simulink model "eVTOL_3DVisuals"  (R2024a)
settings: Solver=VariableStepAuto  StartTime=0.0  StopTime=inf  RelTol=1e-3
libraries: etargetslib x3, slrealtimeiplib x3, sim3dlib x1, uavsim3dlib x1, uavutilslib x1
settings Model: DataDictionary=VTOLDynamicsData.sldd  Creator=jatin.anand  LastModifiedBy=jatin.anand

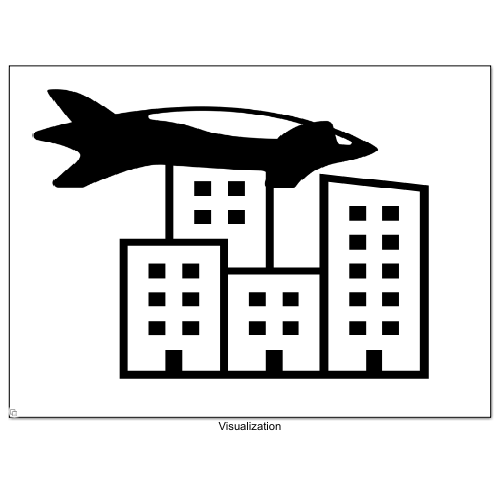
[thumbnail: Simulink's stored preview of the top-level diagram]
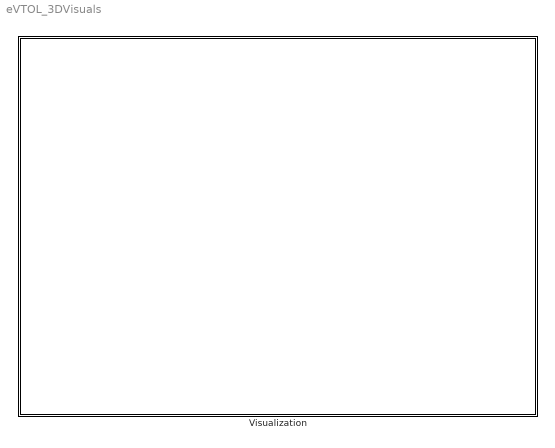
== system eVTOL_3DVisuals ==
  Visualization : Subsystem  Variant=on  VariantControl=Visualization
      mask Display: image('3DVisualization.png');

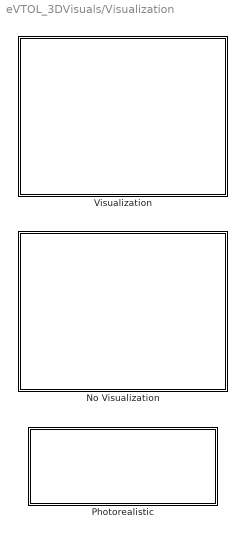
== system eVTOL_3DVisuals/Visualization ==
  No Visualization : Subsystem  VariantControl=Visualization==0
  Photorealistic : Subsystem  VariantControl=Visualization==2
  Visualization : Subsystem  VariantControl=Visualization==1

== system eVTOL_3DVisuals/Visualization/No Visualization ==

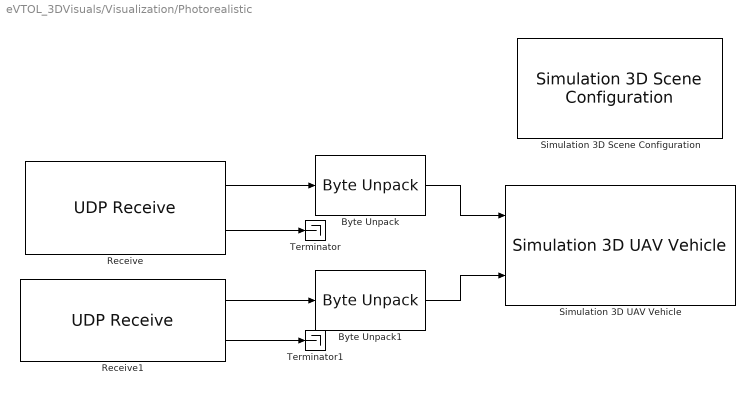
== system eVTOL_3DVisuals/Visualization/Photorealistic ==
  Byte Unpack : etargetslib/Byte Unpack  dimensions={[3]}  datatypes={'double'}  byteAlign=1
      settings: LibrarySourceBlock=embeddedtargetslib/Host Communication/Byte Unpack
  Byte Unpack1 : etargetslib/Byte Unpack  dimensions={[3]}  datatypes={'double'}  byteAlign=1
      settings: LibrarySourceBlock=embeddedtargetslib/Host Communication/Byte Unpack
  Receive : slrealtimeiplib/UDP Receive  useHostTargetConn=on  ipAddress=target_ip  localPort=25002  rcvWidth=24  rcvFmAny=on  fmAddress=host_ip  sampleTime=-1  enableMessage=off  maxPackets=1
  Receive1 : slrealtimeiplib/UDP Receive  useHostTargetConn=on  ipAddress=target_ip  localPort=25003  rcvWidth=24  rcvFmAny=on  fmAddress=host_ip  sampleTime=-1  enableMessage=off  maxPackets=1
  Simulation 3D Scene Configuration : sim3dlib/Simulation 3D Scene Configuration  Priority=0  ProjectFormat=Unreal Editor  SceneDesc=US city block  ProjectName=I:\29\vdubey.MergedFixedWingReview\matlab\toolbox\shared\sim3d_projects\automotive_project_windows\UE\WindowsNoEditor\VehicleSimulation.exe  ScenePath=/Game/Maps/USCityBlock  UEProjPath=C:\project\AutoVrtlEnv\AutoVrtlEnv.uproject  EnableOpenDRIVE=off  vehTagList={'Scene Origin'}  vehTag=Scene Origin  FreeCameraInitialTranslation=[0, 0, 0]  FreeCameraDefaultInitialTranslation=[-6, 0, 2]  FreeCameraInitialRotation=[0, 0, 0]  FreeCameraDefaultInitialRotation=[0, -15, 0]  OpVisEn=off  Ts=1/10  EnableWindow=on  EnableRemoteAccess=off  EnableWeather=off  SunAzimuth=90  SunAltitude=40.0  EnableGeospatialSun=off  Latitude=0  Longitude=0  Date=2023-01-01  Time=10:30:00  GeoTimeZone=-5.0  SunDaylightSaving=off  wind=1  clouds=10  EnableVolumetricClouds=off  CloudCoverage=0  CloudAltitude=6  fog=0  rain=0  RaindropsEffect=off  SnowDensity=0  EnableGeospatial=off  UseTrueOrigin=off  OriginHeight=200  OriginLatitude=40.744652  OriginLongitude=-73.988864  MapStyle=Aerial  AdditionalAssetIDs=[]  UseAdvancedSunSky=off  SolarTime=11  TimeZone=-5  Day=21  Month=9  Year=2022  UseDaylightSavingTime=on  DSTStartDay=10  DSTStartMonth=3  DSTEndDay=3  DSTEndMonth=11  DSTSwitchHour=2  sensorTag=MainCamera1  sensorId=1  sensorName=MainCamera1  mountLoc=Origin  offsetFlag=off  tmountOffset=[0, 0, 0]  rmountOffset=[0, 0, 0]  HorizontalResolution=1280  VerticalResolution=720  HorizontalFOV=60  mountPoint=[0 0 0]  mountOrientation=[0 0 0]  aMode=4  ID=1  GeoTrigger=Inactive
      link override Simulation 3D Engine: SceneDesc=US city block
      settings: LibrarySourceBlock=uavsim3dlib/Simulation 3D Scene Configuration
  Simulation 3D UAV Vehicle : uavsim3dlib/Simulation 3D UAV Vehicle  Priority=-1  Mesh=Custom  MeshPath=SkeletalMesh'/Game/Maps/VTOLDEMO/VTOLAsset.VTOLAsset'  Color=Black  ActorName=SimulinkVehicle1  UseGlobalFrame=off  InitialTranslation=[0 0 0]  InitialRotation=[0 0 0]  InitialTranslationGlobal=[0 0 0]  InitialGeoOrigin=[0 0 0]  InitialRotationGlobal=[0 0 0]  SampleTime=0.1  ActorType=SimulinkVehicle  ID=1  aMode=4  ActorTag=SimulinkVehicle1
  Terminator : Terminator
  Terminator1 : Terminator
  wires:
  Receive1/1 -> Byte Unpack1/1
  Receive/1 -> Byte Unpack/1
  Receive/2 -> Terminator/1
  Receive1/2 -> Terminator1/1
  Byte Unpack/1 -> Simulation 3D UAV Vehicle/1
  Byte Unpack1/1 -> Simulation 3D UAV Vehicle/2

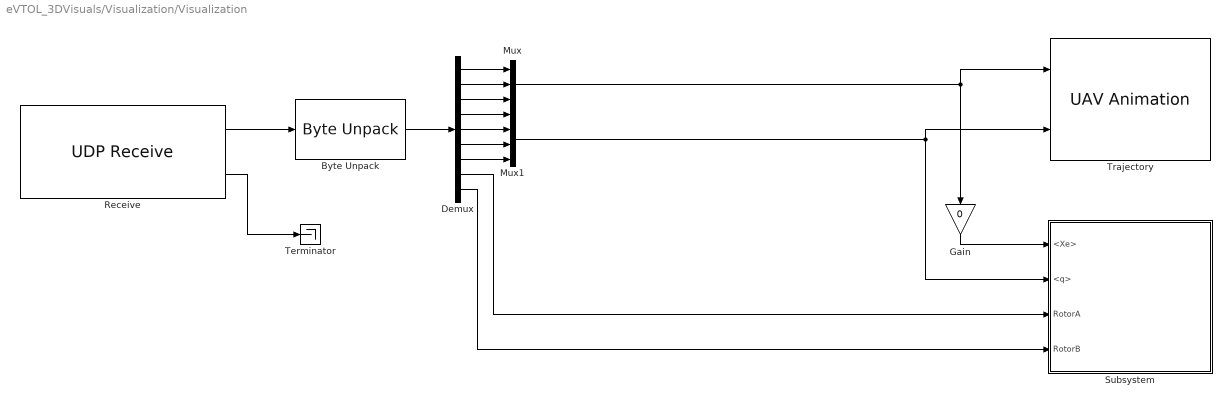
== system eVTOL_3DVisuals/Visualization/Visualization ==
  Byte Unpack : etargetslib/Byte Unpack  dimensions={[9]}  datatypes={'double'}  byteAlign=1
      settings: LibrarySourceBlock=embeddedtargetslib/Host Communication/Byte Unpack
  Demux : Demux  Outputs=9
  Gain : Gain  Gain=0
  Mux : Mux  Inputs=3
  Mux1 : Mux
  Receive : slrealtimeiplib/UDP Receive  useHostTargetConn=on  ipAddress=target_ip  localPort=25002  rcvWidth=72  rcvFmAny=on  fmAddress=host_ip  sampleTime=-1  enableMessage=off  maxPackets=1
  Subsystem : Subsystem
  Terminator : Terminator
  Trajectory : uavutilslib/UAV Animation  UAVType=FixedWing  UAVSize=6  InertialZDirection=Down  SampleTime=0.1
  wires:
  Mux1/1 -> Subsystem/2(<q>), Trajectory/2
  Mux/1 -> Trajectory/1, Gain/1
  Gain/1 -> Subsystem/1(<Xe>)
  Demux/8 -> Subsystem/3(RotorA)
  Demux/9 -> Subsystem/4(RotorB)
  Receive/1 -> Byte Unpack/1
  Byte Unpack/1 -> Demux/1
  Receive/2 -> Terminator/1
  Demux/1 -> Mux/1
  Demux/2 -> Mux/2
  Demux/3 -> Mux/3
  Demux/4 -> Mux1/1
  Demux/5 -> Mux1/2
  Demux/6 -> Mux1/3
  Demux/7 -> Mux1/4

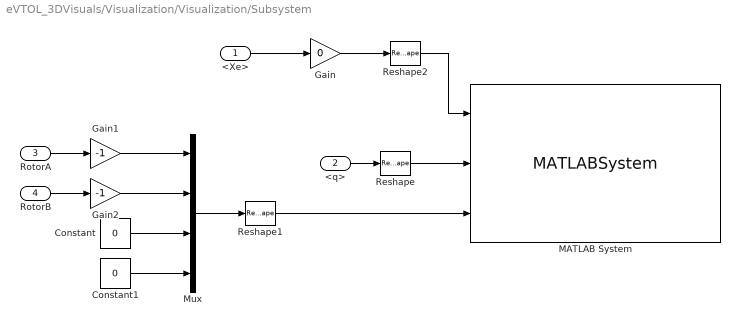
== system eVTOL_3DVisuals/Visualization/Visualization/Subsystem ==
  <Xe> : Inport
  <q> : Inport  Port=2
  RotorA : Inport  Port=3
  RotorB : Inport  Port=4
  Constant : Constant  Value=0
  Constant1 : Constant  Value=0
  Gain : Gain  Gain=0
  Gain1 : Gain  Gain=-1
  Gain2 : Gain  Gain=-1
  MATLAB System : MATLABSystem  System=exampleHelperTiltRotorAnimator  SampleTime=0.05
      mask Type: exampleHelperTiltRotorAnimator
      mask Display:
      | disp('exampleHelperTiltRotorAnimator');
      | port_label('input',1,'position');
      | port_label('input',2,'orientation');
      | port_label('input',3,'rotorAngles');
  Mux : Mux
  Reshape : Reshape  OutputDimensionality=Customize  OutputDimensions=[1,4]
  Reshape1 : Reshape  OutputDimensionality=Customize  OutputDimensions=[1,4]
  Reshape2 : Reshape  OutputDimensionality=Customize  OutputDimensions=[1,3]
  wires:
  Gain1/1 -> Mux/1
  Constant1/1 -> Mux/4
  Gain2/1 -> Mux/2
  Reshape1/1 -> MATLAB System/3
  Mux/1 -> Reshape1/1
  RotorA/1 -> Gain1/1
  <Xe>/1 -> Gain/1
  Constant/1 -> Mux/3
  RotorB/1 -> Gain2/1
  <q>/1 -> Reshape/1
  Reshape2/1 -> MATLAB System/1
  Reshape/1 -> MATLAB System/2
  Gain/1 -> Reshape2/1
